simulink model "W06_Tiny_Town_cs"  (R2019a)
settings: Solver=ode5  StartTime=0.0  StopTime=inf  FixedStep=1/20  RelTol=1e-3
PreLoadFcn:
  | mbxruntime.callbacks.PreLoadFcn(bdroot);
PostLoadFcn:
  | mbxruntime.callbacks.PostLoadFcn(bdroot);
InitFcn:
  | mbxruntime.callbacks.InitFcn(bdroot);
StartFcn:
  | mbxruntime.callbacks.StartFcn(bdroot);
StopFcn:
  | mbxruntime.callbacks.StopFcn(bdroot);
model workspace: external: MAT-File .\W06_Tiny_Town_cs_hws.mat (data not in the file)
undefined symbols (not defined in the file or in its folder): DiscIntNeverNeededParam, InitImageOutputDir, mbxruntime, tabledata, W06_Tiny_Town_cs_0347f368afc477f7, W06_Tiny_Town_cs_06d739b3240d4bd1, W06_Tiny_Town_cs_0f8ec0220805dc92, W06_Tiny_Town_cs_158eea2914cd8c14, W06_Tiny_Town_cs_18b17a0c58606dc8, W06_Tiny_Town_cs_19806d8538d6bb90, W06_Tiny_Town_cs_1ceb610c831ebc6c, W06_Tiny_Town_cs_24c71a941f2399ee, W06_Tiny_Town_cs_28d17e17e50ff375, W06_Tiny_Town_cs_29e44574efa0e72f, W06_Tiny_Town_cs_2ebfd9727ae5049f, W06_Tiny_Town_cs_3b9dd96920beca23, W06_Tiny_Town_cs_4a5ba1a10aa72aa4, W06_Tiny_Town_cs_4b7992cae6b11fea, W06_Tiny_Town_cs_4ce1089559374df3, W06_Tiny_Town_cs_4f1eca6f5670696f, W06_Tiny_Town_cs_56de7514e81a64a4, W06_Tiny_Town_cs_5815099e4ab8d5b1, W06_Tiny_Town_cs_59a193f7803a15f8, W06_Tiny_Town_cs_5a93c0b4041e538b, W06_Tiny_Town_cs_5e22ff2291c0d8f8, W06_Tiny_Town_cs_664a4c8dcb6e1d77, W06_Tiny_Town_cs_66e74ff0a825ce8c, W06_Tiny_Town_cs_6f6fc115e33636b9, W06_Tiny_Town_cs_762b24f74e6359cd, W06_Tiny_Town_cs_7e7dfe0ad6d20cde, W06_Tiny_Town_cs_8dbb769f58f1ae22, W06_Tiny_Town_cs_9732a70429881892, W06_Tiny_Town_cs_97e2037932c1d396, W06_Tiny_Town_cs_99e9b9fe56cd6c11, W06_Tiny_Town_cs_9d4b19fadf9db3f5, W06_Tiny_Town_cs_9e5d5712939b904c, W06_Tiny_Town_cs_9fe5ad465f6cdbf3, W06_Tiny_Town_cs_a263437ac60b94d3, W06_Tiny_Town_cs_a313ed4746bdbf42, W06_Tiny_Town_cs_a3bc7bd64557c06d, W06_Tiny_Town_cs_af25170a5cd54ac4, W06_Tiny_Town_cs_b0bfde99f178c69e, W06_Tiny_Town_cs_b828188f0394b7ed, W06_Tiny_Town_cs_b8ac5a8063403724, W06_Tiny_Town_cs_c0c1ce03c301d04b, W06_Tiny_Town_cs_c5d7b9713d9c4410, W06_Tiny_Town_cs_cce5d3f0bd4fe0dd, W06_Tiny_Town_cs_d4161cd6ae7b274e, W06_Tiny_Town_cs_d7f1a2863608ebc5, W06_Tiny_Town_cs_e07aed9c56d02b7c, W06_Tiny_Town_cs_e4fcf49468faab60, W06_Tiny_Town_cs_e81ada3a1b2b4b0f, W06_Tiny_Town_cs_f328760c8f041e3e, W06_Tiny_Town_cs_fbbe35eb7fc27d63, W06_Tiny_Town_cs_fe7173e9daa72ca4, W06_Tiny_Town_cs_Female_Regular_1_Path_pathUniqueID, W06_Tiny_Town_cs_Ford_Focus_Stationwagon_2_Path_pathUniqueID, W06_Tiny_Town_cs_Nissan_Cabstar_Boxtruck_1_Path_pathUniqueID
libraries: adeye_lib x38, PreScanSimulinkLibrary x16, simulink x4, simulink_extras x3, robotlib x1, PreScanUsefulBlocks x1
(part 2 of 8)

== system W06_Tiny_Town_cs/ANIM_Child_Regular_1 ==
  ANIM_Child_Regular_1 : Inport  Tag=inport/AnimationOutport  OutDataTypeStr=Bus: PRESCAN_ANIMACTUATORDATA  PortDimensions=1  SampleTime=1/20  BusOutputAsStruct=on
  Actuator : S-Function  FunctionName=sfun_AnimActuator  Parameters=UniqueID, TimeStep  SFunctionDeploymentMode=off  EnableBusSupport=off  mask(PreScan Sink Block: State Animation){UniqueID=28581, TimeStep=1/20}
      mask prompts: UniqueID "Auto-Assigned: Unique ID"; TimeStep "Auto-Assigned: Upload Period [s]"
      mask help: The Human Animation port allows the human to walk, run or bend
      mask Help: eval('openHelp(239)')
      mask Display: image(imread('HumanAnimated.jpg'))
  wires:
  ANIM_Child_Regular_1/1 -> Actuator/1

== system W06_Tiny_Town_cs/ANIM_Female_Regular_1 ==
  ANIM_Female_Regular_1 : Inport  Tag=inport/AnimationOutport  OutDataTypeStr=Bus: PRESCAN_ANIMACTUATORDATA  PortDimensions=1  SampleTime=1/20  BusOutputAsStruct=on
  Actuator : S-Function  FunctionName=sfun_AnimActuator  Parameters=UniqueID, TimeStep  SFunctionDeploymentMode=off  EnableBusSupport=off  mask(PreScan Sink Block: State Animation){UniqueID=28708, TimeStep=1/20}
      mask prompts: UniqueID "Auto-Assigned: Unique ID"; TimeStep "Auto-Assigned: Upload Period [s]"
      mask help: The Human Animation port allows the human to walk, run or bend
      mask Help: eval('openHelp(239)')
      mask Display: image(imread('HumanAnimated.jpg'))
  wires:
  ANIM_Female_Regular_1/1 -> Actuator/1

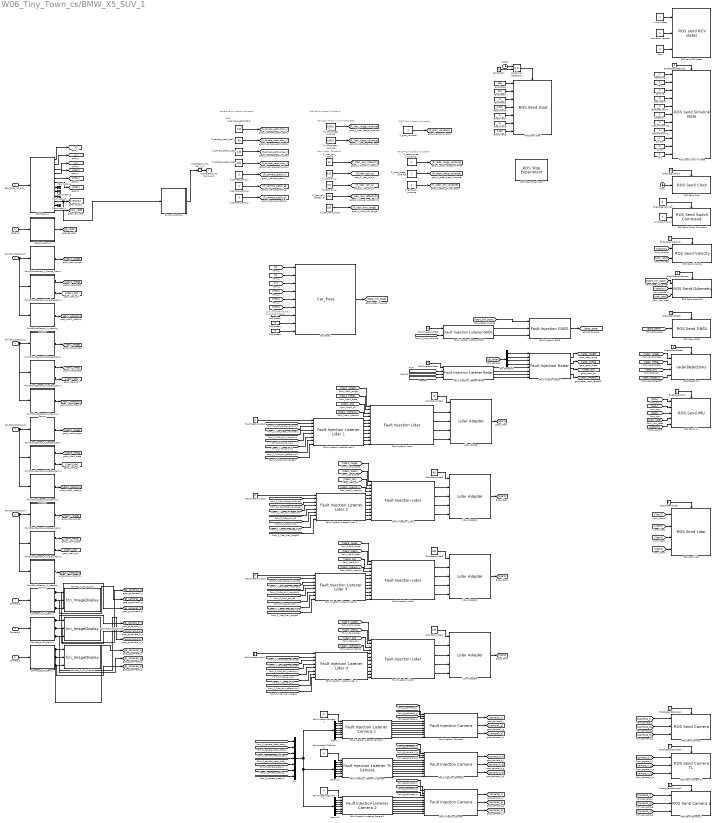
== system W06_Tiny_Town_cs/BMW_X5_SUV_1 ==
  note: CoG  compared
      | to the backwheels
      | center
  note: Gaussian random noise, Parameters
  note: Radar Fault Injection Constants
  note: GNSS Fault Injection Constants
  note: Rain model, Constants
  note: Lidar Fault injection Constants
  note: Patch
  note: Camera Fault injection Constants
  SELF_BMW_X5_SUV_1 : Inport  Tag=inport/SelfPort  OutDataTypeStr=Bus: PRESCAN_SELFSENSORDATA  PortDimensions=1  SampleTime=1/20  BusOutputAsStruct=on
  Radar_1 : Inport  Tag=inport/Radar  Port=2  OutDataTypeStr=Bus: PRESCAN_SCANNERSENSOR_MESSAGE  PortDimensions=7  SampleTime=1/20  BusOutputAsStruct=on
  PointCloudSensor_1 : Inport  Tag=inport/PointCloudInport  Port=3  OutDataTypeStr=single  SampleTime=1/20  BusOutputAsStruct=on
  PointCloudSensor_2 : Inport  Tag=inport/PointCloudInport  Port=4  OutDataTypeStr=single  SampleTime=1/20  BusOutputAsStruct=on
  PointCloudSensor_3 : Inport  Tag=inport/PointCloudInport  Port=5  OutDataTypeStr=single  SampleTime=1/20  BusOutputAsStruct=on
  PointCloudSensor_4 : Inport  Tag=inport/PointCloudInport  Port=6  OutDataTypeStr=single  SampleTime=1/20  BusOutputAsStruct=on
  Camera_1 : Inport  Tag=inport/Camera/CameraSensor  Port=7  OutDataTypeStr=uint8  SampleTime=1/20  BusOutputAsStruct=on
  Camera_tl : Inport  Tag=inport/Camera/CameraSensor  Port=8  OutDataTypeStr=uint8  SampleTime=1/20  BusOutputAsStruct=on
  Camera_2 : Inport  Tag=inport/Camera/CameraSensor  Port=9  OutDataTypeStr=uint8  SampleTime=1/20  BusOutputAsStruct=on
  Activation request : Constant  OutDataTypeStr=Inherit: Inherit via back propagation
  Bus Selector1 : BusSelector  OutputSignals=Range[m],Theta[deg],Phi[deg],TargetTypeID[-]
  Camera_1_CM_Demux : Subsystem  Tag=demux/Camera/Color  mask{SensorName=Camera_1, hres=960, vres=720}
      mask prompts: SensorName "Sensor Name"; hres "Horizontal Resolution"; vres "Vertical Resolution"
      mask Help: eval('openHelp(457)')
      mask Display:
      | fprintf('MONO CAMERA:\n Color\n %s \n %d x %d px',SensorName,hres,vres)
      | port_label('output',1,'R')
      | port_label('output',2,'G')
      | port_label('output',3,'B')
  Camera_1_CM_Display : M-S-Function  Tag=CameraSensor_Color_Display  InitFcn=InitImageOutputDir(gcb);  FunctionName=fcn_ImageDisplay  Parameters=SensorName EnableDisplay EnablePosition DisplayPosition FigureHandle SaveResults BitmapFormat TempOutputDir CameraType DataType  mask(PreScan Color Display Block){SensorName=Camera_1, EnableDisplay=off, EnablePosition=off, DisplayPosition=[10 10 960 720], FigureHandle=2792805, SaveResults=off, Format=PNG, TempOutputDir=0, CameraType=Mono, DataType=uint8}
      mask prompts: SensorName "User Specified: Title of Display"; EnableDisplay "Active"; EnablePosition "Set Display window position"; DisplayPosition "Display window position [xpos ypos width height]"; FigureHandle "Unique Handle"; SaveResults "Save results"; TempOutputDir "OutputDir"; CameraType "Camera Type"; DataType "Image Data Type"
      mask help: This block displays the RGB output of a PreScan camera sensor.
      mask init:
      | if EnableDisplay
      |     EnableString='';
      |     EnableColor='gray';
      | else
      |     EnableString='INACTIVE';
      |     EnableColor='red';
      | end
      | switch Format
      |     case 1
      |         BitmapFormat = 'png';
      |     case 2
      |         BitmapFormat = 'bmp';
      |     case 3
      |         BitmapFormat = 'jpg';
      | end 
      | if CameraType==1
      |     CameraTypeName='MONO';
      |     PortNumber=0;
      | else
      |     CameraTypeName='STEREO';
      |     PortNumber=3;
      | end
      settings: CopyFcn=CopyFcnDisplay  DeleteFcn=PreScanBlockDeleteFcn;  ModelCloseFcn=fcn_ImageDisplay_ModelCloseFcn
      mask Help: eval('openHelp(457)')
      mask Callback EnablePosition:
      | MV=get_param(gcb,'MaskVisibilities');
      | if strcmp(get_param(gcb,'EnablePosition'),'on')
      |     MV{4}='on';
      | else
      |     MV{4}='off';
      | end
      | set_param(gcb,'MaskVisibilities',MV);
      | clear MV;
      mask TypeOptions Format: PNG | BMP | JPG
      mask TypeOptions CameraType: Mono | Stereo
      mask TypeOptions DataType: uint8 | single
      mask Display:
      | color(EnableColor);
      | fprintf('%s\n DISPLAY:\n Color \n %s',EnableString,SensorName)
      | port_label('input',1,'R')
      | port_label('input',2,'G')
      | port_label('input',3,'B')
      | port_label('input',PortNumber+1,'R')
      | port_label('input',PortNumber+2,'G')
      | port_label('input',PortNumber+3,'B')
  Camera_2_CM_Demux : Subsystem  Tag=demux/Camera/Color  mask{SensorName=Camera_2, hres=960, vres=720}
      mask prompts: SensorName "Sensor Name"; hres "Horizontal Resolution"; vres "Vertical Resolution"
      mask Help: eval('openHelp(457)')
      mask Display:
      | fprintf('MONO CAMERA:\n Color\n %s \n %d x %d px',SensorName,hres,vres)
      | port_label('output',1,'R')
      | port_label('output',2,'G')
      | port_label('output',3,'B')
  Camera_2_CM_Display : M-S-Function  Tag=CameraSensor_Color_Display  InitFcn=InitImageOutputDir(gcb);  FunctionName=fcn_ImageDisplay  Parameters=SensorName EnableDisplay EnablePosition DisplayPosition FigureHandle SaveResults BitmapFormat TempOutputDir CameraType DataType  mask(PreScan Color Display Block){SensorName=Camera_2, EnableDisplay=off, EnablePosition=off, DisplayPosition=[10 10 960 720], FigureHandle=2792807, SaveResults=off, Format=PNG, TempOutputDir=0, CameraType=Mono, DataType=uint8}
      mask prompts: SensorName "User Specified: Title of Display"; EnableDisplay "Active"; EnablePosition "Set Display window position"; DisplayPosition "Display window position [xpos ypos width height]"; FigureHandle "Unique Handle"; SaveResults "Save results"; TempOutputDir "OutputDir"; CameraType "Camera Type"; DataType "Image Data Type"
      mask help: This block displays the RGB output of a PreScan camera sensor.
      mask init: same as W06_Tiny_Town_cs/BMW_X5_SUV_1/Camera_1_CM_Display
      settings: CopyFcn=CopyFcnDisplay  DeleteFcn=PreScanBlockDeleteFcn;  ModelCloseFcn=fcn_ImageDisplay_ModelCloseFcn
      mask Help: eval('openHelp(457)')
      mask Callback EnablePosition:
      | MV=get_param(gcb,'MaskVisibilities');
      | if strcmp(get_param(gcb,'EnablePosition'),'on')
      |     MV{4}='on';
      | else
      |     MV{4}='off';
      | end
      | set_param(gcb,'MaskVisibilities',MV);
      | clear MV;
      mask TypeOptions Format: PNG | BMP | JPG
      mask TypeOptions CameraType: Mono | Stereo
      mask TypeOptions DataType: uint8 | single
      mask Display:
      | color(EnableColor);
      | fprintf('%s\n DISPLAY:\n Color \n %s',EnableString,SensorName)
      | port_label('input',1,'R')
      | port_label('input',2,'G')
      | port_label('input',3,'B')
      | port_label('input',PortNumber+1,'R')
      | port_label('input',PortNumber+2,'G')
      | port_label('input',PortNumber+3,'B')
  Camera_tl_CM_Demux : Subsystem  Tag=demux/Camera/Color  mask{SensorName=Camera_tl, hres=960, vres=720}
      mask prompts: SensorName "Sensor Name"; hres "Horizontal Resolution"; vres "Vertical Resolution"
      mask Help: eval('openHelp(457)')
      mask Display:
      | fprintf('MONO CAMERA:\n Color\n %s \n %d x %d px',SensorName,hres,vres)
      | port_label('output',1,'R')
      | port_label('output',2,'G')
      | port_label('output',3,'B')
  Camera_tl_CM_Display : M-S-Function  Tag=CameraSensor_Color_Display  InitFcn=InitImageOutputDir(gcb);  FunctionName=fcn_ImageDisplay  Parameters=SensorName EnableDisplay EnablePosition DisplayPosition FigureHandle SaveResults BitmapFormat TempOutputDir CameraType DataType  mask(PreScan Color Display Block){SensorName=Camera_tl, EnableDisplay=off, EnablePosition=off, DisplayPosition=[10 10 960 720], FigureHandle=2792806, SaveResults=off, Format=PNG, TempOutputDir=0, CameraType=Mono, DataType=uint8}
      mask prompts: SensorName "User Specified: Title of Display"; EnableDisplay "Active"; EnablePosition "Set Display window position"; DisplayPosition "Display window position [xpos ypos width height]"; FigureHandle "Unique Handle"; SaveResults "Save results"; TempOutputDir "OutputDir"; CameraType "Camera Type"; DataType "Image Data Type"
      mask help: This block displays the RGB output of a PreScan camera sensor.
      mask init: same as W06_Tiny_Town_cs/BMW_X5_SUV_1/Camera_1_CM_Display
      settings: CopyFcn=CopyFcnDisplay  DeleteFcn=PreScanBlockDeleteFcn;  ModelCloseFcn=fcn_ImageDisplay_ModelCloseFcn
      mask Help: eval('openHelp(457)')
      mask Callback EnablePosition:
      | MV=get_param(gcb,'MaskVisibilities');
      | if strcmp(get_param(gcb,'EnablePosition'),'on')
      |     MV{4}='on';
      | else
      |     MV{4}='off';
      | end
      | set_param(gcb,'MaskVisibilities',MV);
      | clear MV;
      mask TypeOptions Format: PNG | BMP | JPG
      mask TypeOptions CameraType: Mono | Stereo
      mask TypeOptions DataType: uint8 | single
      mask Display:
      | color(EnableColor);
      | fprintf('%s\n DISPLAY:\n Color \n %s',EnableString,SensorName)
      | port_label('input',1,'R')
      | port_label('input',2,'G')
      | port_label('input',3,'B')
      | port_label('input',PortNumber+1,'R')
      | port_label('input',PortNumber+2,'G')
      | port_label('input',PortNumber+3,'B')
  Car_Pose1 : adeye_lib/Car_Pose  SystemSampleTime=-1
  Clock : Clock
  Clock2 : Clock
  CoG offset x : Constant  Value=0
  CoG offset y : Constant  Value=0
  CoG offset z : Constant  Value=0
  Constant27 : Constant  Value=0
  Demux : Demux  Outputs=7
  Demux1 : Demux  Outputs=7
  Demux2 : Demux  Outputs=7
  Detection : Constant
  Dynamics_Empty : Subsystem  Tag=Dynamics_Empty
      mask Help: eval('openHelp(202)')
      mask Display: port_label('output', 1, 'State');text(0,0,' Empty\n')
  EnableSendCamera1 : Constant  OutDataTypeStr=Inherit: Inherit via back propagation
  EnableSendCamera2 : Constant  OutDataTypeStr=Inherit: Inherit via back propagation
  EnableSendCameraTL : Constant  OutDataTypeStr=Inherit: Inherit via back propagation
  EnableSendClock : Constant  OutDataTypeStr=Inherit: Inherit via back propagation
  EnableSendFeatures : Constant  Value=0  OutDataTypeStr=Inherit: Inherit via back propagation
  EnableSendGNSS : Constant  OutDataTypeStr=Inherit: Inherit via back propagation
  EnableSendIMU : Constant  OutDataTypeStr=Inherit: Inherit via back propagation
  EnableSendLidar : Constant  OutDataTypeStr=Inherit: Inherit via back propagation
  EnableSendOdometry : Constant
  EnableSendRadar : Constant  OutDataTypeStr=Inherit: Inherit via back propagation
  EnableSendSwitch : Constant  Value=0  OutDataTypeStr=Inherit: Inherit via back propagation  SampleTime=0.05
  EnableSendVelocity : Constant  OutDataTypeStr=Inherit: Inherit via back propagation
  FakeLocalization : Constant
  Fault : Constant  Value=0  OutDataTypeStr=Inherit: Inherit via back propagation
  Fault Injection Camera : adeye_lib/Fault Injection Camera  idy=200  idx=100  x=100  y=150  R=0  G=0  B=0
  Fault Injection Camera1 : adeye_lib/Fault Injection Camera  idy=200  idx=100  x=100  y=150  R=0  G=0  B=0
  Fault Injection Camera2 : adeye_lib/Fault Injection Camera  idy=200  idx=100  x=100  y=150  R=0  G=0  B=0
  Fault Injection GNSS : adeye_lib/Fault Injection GNSS  f=20
  Fault Injection Lidar{,1..3} (4 alike) : adeye_lib/Fault Injection Lidar  f=20  p=225*16
  Fault Injection Listener Camera 1 : adeye_lib/Fault Injection Listener Camera 1  SystemSampleTime=-1
  Fault Injection Listener Camera 2 : adeye_lib/Fault Injection Listener Camera 2  SystemSampleTime=-1
  Fault Injection Listener GNSS : adeye_lib/Fault Injection Listener GNSS  SystemSampleTime=-1
  Fault Injection Listener Lidar 1 : adeye_lib/Fault Injection Listener Lidar 1  SystemSampleTime=-1
  Fault Injection Listener Lidar 2 : adeye_lib/Fault Injection Listener Lidar 2  SystemSampleTime=-1
  Fault Injection Listener Lidar 3 : adeye_lib/Fault Injection Listener Lidar 3  SystemSampleTime=-1
  Fault Injection Listener Lidar 4 : adeye_lib/Fault Injection Listener Lidar 4  SystemSampleTime=-1
  Fault Injection Listener Radar : adeye_lib/Fault Injection Listener Radar  SystemSampleTime=-1
  Fault Injection Listener TL Camera : adeye_lib/Fault Injection Listener TL Camera  SystemSampleTime=-1
  Fault Injection Radar : adeye_lib/Fault Injection Radar  n=7
  FaultInjectionCamera1 : Constant  Value=0
  FaultInjectionCamera2 : Constant  Value=0
  FaultInjectionGNSS : Constant  Value=0  OutDataTypeStr=Inherit: Inherit via back propagation  SampleTime=0.05
  FaultInjectionLidar{1..4} (4 alike) : Constant  Value=0  OutDataTypeStr=Inherit: Inherit via back propagation
  FaultInjectionRadar : Constant  Value=0
  FaultInjectionTLCamera : Constant  Value=0
  GoalOrientW : Constant  Value=0.707
  GoalOrientX : Constant  Value=0
  GoalOrientY : Constant  Value=0
  GoalOrientZ : Constant  Value=0.707
  GoalPoseX : Constant  Value=183
  GoalPoseY : Constant  Value=111
  GoalPoseZ : Constant  Value=0
  Initial checks : Constant  OutDataTypeStr=Inherit: Inherit via back propagation
  Lidar Adapter{,1..3} (4 alike) : adeye_lib/Lidar Adapter  SystemSampleTime=-1
  Localization : Constant  Value=0
  Map : Constant
  MissionPlanning : Constant
  MotionPlanning : Constant
  Mux : Mux  Inputs=7
  OrientationLidar1 : Constant  Value=0  OutDataTypeStr=Inherit: Inherit via back propagation
  OrientationLidar2 : Constant  Value=90  OutDataTypeStr=Inherit: Inherit via back propagation
  OrientationLidar3 : Constant  Value=180  OutDataTypeStr=Inherit: Inherit via back propagation
  OrientationLidar4 : Constant  Value=270  OutDataTypeStr=Inherit: Inherit via back propagation
  PointCloudSensor_1_Angles_Demux : Subsystem  Tag=demux/PCS/Angles  mask{SensorName=PointCloudSensor_1, offset=225, hres=225, vres=16}
      mask prompts: SensorName "Sensor Name"; offset "Data Start"; hres "Horizontal Resolution"; vres "Vertical Resolution"
      mask Help: eval('openHelp(6400)')
      mask Display:
      | fprintf('Point Cloud:\n Data\n %s \n %d x %d px',SensorName,hres,vres)
      | port_label('output',1,'Theta')
      | port_label('output',2,'Phi')
  PointCloudSensor_1_Intensity_Demux : Subsystem  Tag=demux/PCS/Intensity  mask{SensorName=PointCloudSensor_1, offset=675, hres=225, vres=16}
      mask prompts: SensorName "Sensor Name"; offset "Data Start"; hres "Horizontal Resolution"; vres "Vertical Resolution"
      mask Help: eval('openHelp(6400)')
      mask Display:
      | fprintf('Point Cloud:\n Data\n %s \n %d x %d px',SensorName,hres,vres)
      | port_label('output',1,'Intensity')
  PointCloudSensor_1_Range_Demux : Subsystem  Tag=demux/PCS/Range  mask{SensorName=PointCloudSensor_1, offset=0, hres=225, vres=16}
      mask prompts: SensorName "Sensor Name"; offset "Data Start"; hres "Horizontal Resolution"; vres "Vertical Resolution"
      mask Help: eval('openHelp(6400)')
      mask Display:
      | fprintf('Point Cloud:\n Data\n %s \n %d x %d px',SensorName,hres,vres)
      | port_label('output',1,'Range')
  PointCloudSensor_2_Angles_Demux : Subsystem  Tag=demux/PCS/Angles  mask{SensorName=PointCloudSensor_2, offset=225, hres=225, vres=16}
      mask prompts: SensorName "Sensor Name"; offset "Data Start"; hres "Horizontal Resolution"; vres "Vertical Resolution"
      mask Help: eval('openHelp(6400)')
      mask Display:
      | fprintf('Point Cloud:\n Data\n %s \n %d x %d px',SensorName,hres,vres)
      | port_label('output',1,'Theta')
      | port_label('output',2,'Phi')
  PointCloudSensor_2_Intensity_Demux : Subsystem  Tag=demux/PCS/Intensity  mask{SensorName=PointCloudSensor_2, offset=675, hres=225, vres=16}
      mask prompts: SensorName "Sensor Name"; offset "Data Start"; hres "Horizontal Resolution"; vres "Vertical Resolution"
      mask Help: eval('openHelp(6400)')
      mask Display:
      | fprintf('Point Cloud:\n Data\n %s \n %d x %d px',SensorName,hres,vres)
      | port_label('output',1,'Intensity')
  PointCloudSensor_2_Range_Demux : Subsystem  Tag=demux/PCS/Range  mask{SensorName=PointCloudSensor_2, offset=0, hres=225, vres=16}
      mask prompts: SensorName "Sensor Name"; offset "Data Start"; hres "Horizontal Resolution"; vres "Vertical Resolution"
      mask Help: eval('openHelp(6400)')
      mask Display:
      | fprintf('Point Cloud:\n Data\n %s \n %d x %d px',SensorName,hres,vres)
      | port_label('output',1,'Range')
  PointCloudSensor_3_Angles_Demux : Subsystem  Tag=demux/PCS/Angles  mask{SensorName=PointCloudSensor_3, offset=225, hres=225, vres=16}
      mask prompts: SensorName "Sensor Name"; offset "Data Start"; hres "Horizontal Resolution"; vres "Vertical Resolution"
      mask Help: eval('openHelp(6400)')
      mask Display:
      | fprintf('Point Cloud:\n Data\n %s \n %d x %d px',SensorName,hres,vres)
      | port_label('output',1,'Theta')
      | port_label('output',2,'Phi')
  PointCloudSensor_3_Intensity_Demux : Subsystem  Tag=demux/PCS/Intensity  mask{SensorName=PointCloudSensor_3, offset=675, hres=225, vres=16}
      mask prompts: SensorName "Sensor Name"; offset "Data Start"; hres "Horizontal Resolution"; vres "Vertical Resolution"
      mask Help: eval('openHelp(6400)')
      mask Display:
      | fprintf('Point Cloud:\n Data\n %s \n %d x %d px',SensorName,hres,vres)
      | port_label('output',1,'Intensity')
  PointCloudSensor_3_Range_Demux : Subsystem  Tag=demux/PCS/Range  mask{SensorName=PointCloudSensor_3, offset=0, hres=225, vres=16}
      mask prompts: SensorName "Sensor Name"; offset "Data Start"; hres "Horizontal Resolution"; vres "Vertical Resolution"
      mask Help: eval('openHelp(6400)')
      mask Display:
      | fprintf('Point Cloud:\n Data\n %s \n %d x %d px',SensorName,hres,vres)
      | port_label('output',1,'Range')
  PointCloudSensor_4_Angles_Demux : Subsystem  Tag=demux/PCS/Angles  mask{SensorName=PointCloudSensor_4, offset=225, hres=225, vres=16}
      mask prompts: SensorName "Sensor Name"; offset "Data Start"; hres "Horizontal Resolution"; vres "Vertical Resolution"
      mask Help: eval('openHelp(6400)')
      mask Display:
      | fprintf('Point Cloud:\n Data\n %s \n %d x %d px',SensorName,hres,vres)
      | port_label('output',1,'Theta')
      | port_label('output',2,'Phi')
  PointCloudSensor_4_Intensity_Demux : Subsystem  Tag=demux/PCS/Intensity  mask{SensorName=PointCloudSensor_4, offset=675, hres=225, vres=16}
      mask prompts: SensorName "Sensor Name"; offset "Data Start"; hres "Horizontal Resolution"; vres "Vertical Resolution"
      mask Help: eval('openHelp(6400)')
      mask Display:
      | fprintf('Point Cloud:\n Data\n %s \n %d x %d px',SensorName,hres,vres)
      | port_label('output',1,'Intensity')
  PointCloudSensor_4_Range_Demux : Subsystem  Tag=demux/PCS/Range  mask{SensorName=PointCloudSensor_4, offset=0, hres=225, vres=16}
      mask prompts: SensorName "Sensor Name"; offset "Data Start"; hres "Horizontal Resolution"; vres "Vertical Resolution"
      mask Help: eval('openHelp(6400)')
      mask Display:
      | fprintf('Point Cloud:\n Data\n %s \n %d x %d px',SensorName,hres,vres)
      | port_label('output',1,'Range')
  ROS Send Camera : adeye_lib/ROS Send Camera  SystemSampleTime=-1
  ROS Send Camera 2 : adeye_lib/ROS Send Camera 2  SystemSampleTime=-1
  ROS Send Camera TL : adeye_lib/ROS Send Camera TL  SystemSampleTime=-1
  ROS Send Clock : adeye_lib/ROS Send Clock  SystemSampleTime=-1
  ROS Send GNSS : adeye_lib/ROS Send GNSS  SystemSampleTime=-1
  ROS Send Goal : adeye_lib/ROS Send Goal  SystemSampleTime=-1
  ROS Send IMU : adeye_lib/ROS Send IMU  SystemSampleTime=-1
  ROS Send Lidar : adeye_lib/ROS Send Lidar  SystemSampleTime=-1
  ROS Send Odometry : adeye_lib/ROS Send Odometry  SystemSampleTime=-1
  ROS Send Simulink State : adeye_lib/ROS Send Simulink State  SystemSampleTime=-1
  ROS Send Switch Command : adeye_lib/ROS Send Switch Command  SystemSampleTime=-1
  ROS Send Velocity : adeye_lib/ROS Send Velocity  SystemSampleTime=-1
  "ROS Stop Experiment " : adeye_lib/ROS Stop Experiment  SystemSampleTime=-1
  ROS send RCV states : adeye_lib/ROS send RCV states  SystemSampleTime=-1
  Radar_1_Demux : Subsystem  Tag=demux/Radar  TreatAsAtomicUnit=on  mask(PreScan Demux Block: Radar){MAXMESSAGES=7}
      mask prompts: MAXMESSAGES "Number of Objects"
      mask help:
      | The Radar Sensor is a detailed sensor based on a physical radar
      | model that includes Antenna GAIN Maps (AGM) and atmospheric
      | attenuation.
      |
      | For more information, please click Help.
      mask Help: eval('openHelp(1464)')
      mask Display:
      | port_label('input',1,'Radar')
      | port_label('output',1,'Radar Data')
  Recording : Constant
  Relational Operator1 : RelationalOperator  Operator===  OutDataTypeStr=boolean  RndMeth=Simplest
  Rviz : Constant
  SELF_Demux : Subsystem  Tag=demux/SelfPort  mask(PreScan Demux Block:){}
      mask help:
      | The SELF port shows (state) information of the actor itself. The outputs are position in the experiment's axis system and the GPS coordinates, and the object's absolute velocity and compass heading.
      |
      | For more information, please click Help.
      settings: DeleteFcn=PreScanBlockDeleteFcn;
      mask Help: eval('openHelp(462)')
      mask Display:
      | port_label('output',1,'x [m]')
      | port_label('output',2,'y [m]')
      | port_label('output',3,'z [m]','texmode','on')
      | port_label('output',4,'Rotx [deg]','texmode','on')
      | port_label('output',5,'Roty [deg]','texmode','on')
      | port_label('output',6,'Rotz [deg]','texmode','on')
      | port_label('output',7,'GPS lat [deg]','texmode','on')
      | port_label('output',8,'GPS long [deg]','texmode','on')
      | port_label('output',9,'GPS alt [m]','texmode','on')
      | port_label('output',10,'Velocity [m/s]')
      | port_label('output',11,'Heading [deg]')
      | port_label('output',12,'Yaw rate [deg/s]')
  STATE_BMW_X5_SUV_1_rc : RateTransition  Tag=mux_rc/StatePort  OutPortSampleTimeOpt=Inherit
  Sensing : Constant
  Ssmp : Constant
  Switch : Constant
  SwitchCommand : Constant  OutDataTypeStr=Inherit: Inherit via back propagation  SampleTime=0.05
  Terminator_{1..4} (4 alike) : Terminator
  fi_camera_patch_b : Constant  Value=0
  fi_camera_patch_g : Constant  Value=0
  fi_camera_patch_r : Constant  Value=0
  fi_camera_patch_size_x : Constant  Value=100
  fi_camera_patch_size_y : Constant  Value=100
  fi_camera_patch_start_x : Constant  Value=110
  fi_camera_patch_start_y : Constant  Value=50
  fi_gnss_variance : Constant
  fi_lidar_max_range : Constant  Value=150
  fi_lidar_rain_a : Constant  Value=0.01
  fi_lidar_rain_b : Constant  Value=0.6
  fi_lidar_rain_intensity : Constant  Value=20
  fi_lidar_rain_reflectivity : Constant  Value=0.9
  fi_lidar_range_variance : Constant  Value=0.0001
  fi_lidar_theta_variance : Constant  Value=0.0001
  fi_radar_phi_variance : Constant
  fi_radar_range_variance : Constant
  fi_radar_theta_variance : Constant
  radarDetections : adeye_lib/radarDetections  SystemSampleTime=-1
  STATE_BMW_X5_SUV_1_bus : Outport  Tag=outport/StatePort  OutDataTypeStr=Bus: PRESCAN_STATEACTUATORDATA  PortDimensions=1  SampleTime=1/20
  wires:
  GoalOrientZ/1 -> ROS Send Goal/7
  GoalOrientW/1 -> ROS Send Goal/4
  GoalOrientX/1 -> ROS Send Goal/5
  GoalOrientY/1 -> ROS Send Goal/6
  GoalPoseX/1 -> ROS Send Goal/1
  GoalPoseY/1 -> ROS Send Goal/2
  GoalPoseZ/1 -> ROS Send Goal/3
  Constant27/1 -> Relational Operator1/2
  Relational Operator1/1 -> ROS Send Goal/Enable
  Clock2/1 -> Relational Operator1/1
  Demux1/2 -> Fault Injection Listener TL Camera/3
  fi_lidar_range_variance/1 -> [fi_lidar_range_variance]
  Fault Injection Listener Radar/2 -> Fault Injection Radar/6
  [Rotx] -> ROS Send IMU/1
  [lidar1_theta] -> Fault Injection Lidar/2
  Fault Injection Listener TL Camera/1 -> Fault Injection Camera2/4
  Demux/1 -> Fault Injection Listener Camera 1/2
  [gt_camera1_r] -> Fault Injection Camera1/1
  [fi_lidar_rain_reflectivity] -> Fault Injection Listener Lidar 4/7
  Fault Injection Lidar2/4 -> Lidar Adapter2/5
  Demux2/3 -> Fault Injection Listener Camera 2/4
  Mux/1 -> Demux2/1, Demux1/1, Demux/1
  Demux1/3 -> Fault Injection Listener TL Camera/4
  [lidar4_phi] -> Fault Injection Lidar3/3
  [fi_lidar_rain_b] -> Fault Injection Listener Lidar 3/6
  [gt_camera_tl_g] -> Fault Injection Camera2/2
  Fault Injection Radar/2 -> [radar_theta]
  Demux1/7 -> Fault Injection Listener TL Camera/8
  Fault Injection Camera2/1 -> [camera_tl_r]
  Demux2/7 -> Fault Injection Listener Camera 2/8
  [fi_camera_patch_size_x] -> Mux/3
  Fault Injection Camera1/3 -> [camera1_b]
  Demux/2 -> Fault Injection Listener Camera 1/3
  [fi_gnss_variance] -> Fault Injection Listener GNSS/2
  Demux/4 -> Fault Injection Listener Camera 1/5
  Fault Injection Listener Lidar 4/1 -> Fault Injection Lidar3/5
  OrientationLidar1/1 -> Lidar Adapter/1
  Fault Injection Listener Lidar 3/5 -> Fault Injection Lidar2/9
  Fault Injection Camera2/2 -> [camera_tl_g]
  Fault Injection Listener Lidar 4/2 -> Fault Injection Lidar3/6
  Demux/3 -> Fault Injection Listener Camera 1/4
  Demux1/1 -> Fault Injection Listener TL Camera/2
  Fault Injection Listener Lidar 2/8 -> Fault Injection Lidar1/12
  [camera_tl_r] -> ROS Send Camera TL/1
  Activation request/1 -> ROS send RCV states/2
  [fi_camera_patch_g] -> Mux/6
  Demux/7 -> Fault Injection Listener Camera 1/8
  fi_lidar_theta_variance/1 -> [fi_lidar_theta_variance]
  [fi_lidar_range_variance] -> Fault Injection Listener Lidar 2/2
  EnableSendIMU/1 -> ROS Send IMU/Enable
  Fault Injection Listener TL Camera/7 -> Fault Injection Camera2/10
  Demux2/2 -> Fault Injection Listener Camera 2/3
  Demux2/5 -> Fault Injection Listener Camera 2/6
  [fi_lidar_rain_reflectivity] -> Fault Injection Listener Lidar 1/7
  fi_camera_patch_b/1 -> [fi_camera_patch_b]
  Demux1/5 -> Fault Injection Listener TL Camera/6
  [fi_lidar_theta_variance] -> Fault Injection Listener Lidar 3/3
  Fault Injection Listener Lidar 1/1 -> Fault Injection Lidar/5
  fi_camera_patch_g/1 -> [fi_camera_patch_g]
  OrientationLidar4/1 -> Lidar Adapter3/1
  [fi_camera_patch_start_y] -> Mux/2
  [camera2_g] -> ROS Send Camera 2/2
  [fi_lidar_rain_a] -> Fault Injection Listener Lidar 2/5
  FaultInjectionTLCamera/1 -> Fault Injection Listener TL Camera/1
  [lidar4_theta] -> Fault Injection Lidar3/2
  [fi_camera_patch_start_x] -> Mux/1
  [yaw_rate] -> ROS Send IMU/4
  fi_camera_patch_start_x/1 -> [fi_camera_patch_start_x]
  [fi_lidar_max_range] -> Fault Injection Listener Lidar 4/8
  [radar_range] -> radarDetections/1
  [fi_lidar_rain_intensity] -> Fault Injection Listener Lidar 3/4
  [fi_lidar_rain_intensity] -> Fault Injection Listener Lidar 4/4
  fi_camera_patch_size_x/1 -> [fi_camera_patch_size_x]
  [camera1_r] -> ROS Send Camera/1
  Fault Injection Listener Radar/4 -> Fault Injection Radar/8
  Fault Injection Radar/4 -> [radar_targetID]
  [camera2_r] -> ROS Send Camera 2/1
  fi_radar_phi_variance/1 -> [fi_radar_phi_variance]
  [camera1_b] -> ROS Send Camera/3
  fi_camera_patch_r/1 -> [fi_camera_patch_r]
  Fault Injection Camera1/2 -> [camera1_g]
  [fi_lidar_rain_b] -> Fault Injection Listener Lidar 2/6
  Fault Injection Camera/3 -> [camera2_b]
  [fi_lidar_max_range] -> Fault Injection Listener Lidar 3/8
  Fault Injection Lidar1/4 -> Lidar Adapter1/5
  Fault Injection Camera/2 -> [camera2_g]
  Fault Injection Listener Lidar 3/4 -> Fault Injection Lidar2/8
  Fault Injection Lidar1/2 -> Lidar Adapter1/3
  [gt_radar] -> Bus Selector1/1
  [fi_radar_phi_variance] -> Fault Injection Listener Radar/4
  [camera_tl_g] -> ROS Send Camera TL/2
  Fault Injection Listener Lidar 1/3 -> Fault Injection Lidar/7
  Fault Injection Listener Camera 2/6 -> Fault Injection Camera/9
  EnableSendCameraTL/1 -> ROS Send Camera TL/Enable
  Fault Injection Listener Radar/1 -> Fault Injection Radar/5
  [radar_theta] -> radarDetections/2
  Fault Injection Lidar3/3 -> Lidar Adapter3/4
  Fault Injection Listener Lidar 1/4 -> Fault Injection Lidar/8
  [fi_lidar_rain_b] -> Fault Injection Listener Lidar 4/6
  [radar_phi] -> radarDetections/3
  Fault Injection Listener Lidar 2/7 -> Fault Injection Lidar1/11
  [gnss_pose] -> ROS Send GNSS/1
  Fault Injection Radar/1 -> [radar_range]
  fi_lidar_max_range/1 -> [fi_lidar_max_range]
  Fault Injection Listener Lidar 1/6 -> Fault Injection Lidar/10
  [velocity] -> ROS Send IMU/5
  [camera2_b] -> ROS Send Camera 2/3
  Fault Injection Lidar3/2 -> Lidar Adapter3/3
  Fault Injection Listener Camera 2/7 -> Fault Injection Camera/10
  Fault Injection Listener Lidar 1/2 -> Fault Injection Lidar/6
  [lidar3_phi] -> Fault Injection Lidar2/3
  Fault Injection Listener Camera 2/1 -> Fault Injection Camera/4
  [lidar1_range] -> Fault Injection Lidar/1
  [fi_lidar_theta_variance] -> Fault Injection Listener Lidar 4/3
  Fault Injection Listener Camera 2/2 -> Fault Injection Camera/5
  [lidar3_range] -> Fault Injection Lidar2/1
  [lidar2_range] -> Fault Injection Lidar1/1
  [fi_camera_patch_size_y] -> Mux/4
  [lidar2_theta] -> Fault Injection Lidar1/2
  Fault Injection Listener Lidar 3/2 -> Fault Injection Lidar2/6
  fi_camera_patch_start_y/1 -> [fi_camera_patch_start_y]
  fi_gnss_variance/1 -> [fi_gnss_variance]
  [fi_camera_patch_r] -> Mux/5
  [Rotz] -> ROS Send IMU/3
  CoG offset y/1 -> Car_Pose1/8
  [fi_lidar_rain_a] -> Fault Injection Listener Lidar 4/5
  [lidar2_phi] -> Fault Injection Lidar1/3
  Fault Injection GNSS/1 -> [gnss_pose]
  [lidar2_intensity] -> Fault Injection Lidar1/4
  [lidar4_range] -> Fault Injection Lidar3/1
  [fi_radar_theta_variance] -> Fault Injection Listener Radar/3
  [gt_camera2_g] -> Fault Injection Camera/2
  [gt_camera_tl_b] -> Fault Injection Camera2/3
  Clock/1 -> ROS Send Clock/1
  Fault Injection Listener Lidar 4/3 -> Fault Injection Lidar3/7
  Fault Injection Listener TL Camera/2 -> Fault Injection Camera2/5
  Fault Injection Listener TL Camera/6 -> Fault Injection Camera2/9
  [lidar1_phi] -> Fault Injection Lidar/3
  [lidar1_intensity] -> Fault Injection Lidar/4
  Lidar Adapter1/1 -> [lidar2]
  Demux1/6 -> Fault Injection Listener TL Camera/7
  Fault Injection Listener Camera 1/4 -> Fault Injection Camera1/7
  Fault Injection Camera2/3 -> [camera_tl_b]
  [fi_lidar_max_range] -> Fault Injection Listener Lidar 1/8
  Fault Injection Listener TL Camera/8 -> Fault Injection Camera2/11
  Fault Injection Listener Camera 1/5 -> Fault Injection Camera1/8
  Fault Injection Listener Radar/3 -> Fault Injection Radar/7
  Fault Injection Lidar/1 -> Lidar Adapter/2
  Fault Injection Listener Camera 1/3 -> Fault Injection Camera1/6
  Fault Injection Radar/3 -> [radar_phi]
  [fi_radar_range_variance] -> Fault Injection Listener Radar/2
  Fault Injection Listener Camera 1/7 -> Fault Injection Camera1/10
  fi_radar_range_variance/1 -> [fi_radar_range_variance]
  EnableSendFeatures/1 -> ROS Send Simulink State/Enable
  [fi_lidar_range_variance] -> Fault Injection Listener Lidar 1/2
  Demux2/1 -> Fault Injection Listener Camera 2/2
  [fi_lidar_theta_variance] -> Fault Injection Listener Lidar 1/3
  Fault Injection Listener Lidar 4/7 -> Fault Injection Lidar3/11
  Fault Injection Listener Lidar 3/6 -> Fault Injection Lidar2/10
  Fault Injection Listener Lidar 4/8 -> Fault Injection Lidar3/12
  Fault Injection Listener Lidar 3/3 -> Fault Injection Lidar2/7
  Fault Injection Listener TL Camera/4 -> Fault Injection Camera2/7
  Fault Injection Listener Lidar 3/7 -> Fault Injection Lidar2/11
  Fault Injection Listener Camera 2/8 -> Fault Injection Camera/11
  Fault Injection Listener Lidar 3/8 -> Fault Injection Lidar2/12
  [fi_lidar_rain_intensity] -> Fault Injection Listener Lidar 1/4
  Fault Injection Listener Camera 2/5 -> Fault Injection Camera/8
  Fault Injection Listener Camera 1/8 -> Fault Injection Camera1/11
  Fault Injection Listener TL Camera/3 -> Fault Injection Camera2/6
  OrientationLidar3/1 -> Lidar Adapter2/1
  [fi_camera_patch_b] -> Mux/7
  Fault Injection Listener Camera 2/3 -> Fault Injection Camera/6
  Fault Injection Lidar1/1 -> Lidar Adapter1/2
  Fault Injection Listener Lidar 2/4 -> Fault Injection Lidar1/8
  SwitchCommand/1 -> ROS Send Switch Command/1
  FaultInjectionLidar2/1 -> Fault Injection Listener Lidar 2/1
  [fi_lidar_range_variance] -> Fault Injection Listener Lidar 4/2
  Map/1 -> ROS Send Simulink State/2
  Demux/5 -> Fault Injection Listener Camera 1/6
  Fault Injection Listener Lidar 2/3 -> Fault Injection Lidar1/7
  Fault Injection Lidar1/3 -> Lidar Adapter1/4
  Fault Injection Lidar2/2 -> Lidar Adapter2/3
  Demux2/4 -> Fault Injection Listener Camera 2/5
  Fault Injection Lidar2/3 -> Lidar Adapter2/4
  MissionPlanning/1 -> ROS Send Simulink State/7
  Fault Injection Listener Lidar 3/1 -> Fault Injection Lidar2/5
  [gt_camera1_b] -> Fault Injection Camera1/3
  [gt_camera_tl_r] -> Fault Injection Camera2/1
  [lidar4_intensity] -> Fault Injection Lidar3/4
  [gt_camera1_g] -> Fault Injection Camera1/2
  Ssmp/1 -> ROS Send Simulink State/10
  FaultInjectionCamera2/1 -> Fault Injection Listener Camera 2/1
  Fault Injection Listener Lidar 1/5 -> Fault Injection Lidar/9
  Fault Injection Listener GNSS/2 -> Fault Injection GNSS/3
  Fault Injection Listener Lidar 2/2 -> Fault Injection Lidar1/6
  Demux/6 -> Fault Injection Listener Camera 1/7
  [fi_lidar_rain_a] -> Fault Injection Listener Lidar 1/5
  Fault Injection Listener Lidar 2/1 -> Fault Injection Lidar1/5
  Fault Injection Lidar/4 -> Lidar Adapter/5
  Fault Injection Listener Camera 1/1 -> Fault Injection Camera1/4
  Fault Injection Camera1/1 -> [camera1_r]
  [gt_camera2_b] -> Fault Injection Camera/3
  Fault Injection Camera/1 -> [camera2_r]
  [fi_lidar_rain_b] -> Fault Injection Listener Lidar 1/6
  [yaw_rate] -> ROS Send Velocity/2
  Demux2/6 -> Fault Injection Listener Camera 2/7
  FaultInjectionLidar3/1 -> Fault Injection Listener Lidar 3/1
  FaultInjectionCamera1/1 -> Fault Injection Listener Camera 1/1
  FaultInjectionLidar1/1 -> Fault Injection Listener Lidar 1/1
  Lidar Adapter3/1 -> [lidar4]
  [fi_lidar_range_variance] -> Fault Injection Listener Lidar 3/2
  Recording/1 -> ROS Send Simulink State/1
  MotionPlanning/1 -> ROS Send Simulink State/8
  FaultInjectionGNSS/1 -> Fault Injection Listener GNSS/1
  fi_lidar_rain_a/1 -> [fi_lidar_rain_a]
  fi_lidar_rain_reflectivity/1 -> [fi_lidar_rain_reflectivity]
  FakeLocalization/1 -> ROS Send Simulink State/5
  EnableSendVelocity/1 -> ROS Send Velocity/Enable
  FaultInjectionLidar4/1 -> Fault Injection Listener Lidar 4/1
  [lidar2] -> ROS Send Lidar/2
  [lidar4] -> ROS Send Lidar/4
  EnableSendCamera2/1 -> ROS Send Camera 2/Enable
  Fault Injection Listener TL Camera/5 -> Fault Injection Camera2/8
  [base_link_pose] -> Fault Injection GNSS/1
  EnableSendSwitch/1 -> ROS Send Switch Command/Enable
  EnableSendLidar/1 -> ROS Send Lidar/Enable
  Fault Injection Listener Camera 1/6 -> Fault Injection Camera1/9
  [lidar1] -> ROS Send Lidar/1
  [velocity] -> ROS Send Velocity/1
  Fault Injection Listener Lidar 4/5 -> Fault Injection Lidar3/9
  Initial checks/1 -> ROS send RCV states/1
  CoG offset z/1 -> Car_Pose1/9
  Switch/1 -> ROS Send Simulink State/9
  EnableSendGNSS/1 -> ROS Send GNSS/Enable
  Demux1/4 -> Fault Injection Listener TL Camera/5
  Fault Injection Lidar/2 -> Lidar Adapter/3
  OrientationLidar2/1 -> Lidar Adapter1/1
  Fault Injection Listener Lidar 2/5 -> Fault Injection Lidar1/9
  [radar_targetID] -> radarDetections/4
  [Roty] -> Car_Pose1/5
  [base_link_pose] -> ROS Send Odometry/1
  [yaw_rate] -> ROS Send Odometry/3
  Fault Injection Listener Lidar 4/6 -> Fault Injection Lidar3/10
  fi_lidar_rain_intensity/1 -> [fi_lidar_rain_intensity]
  Detection/1 -> ROS Send Simulink State/6
  [velocity] -> ROS Send Odometry/2
  EnableSendOdometry/1 -> ROS Send Odometry/Enable
  EnableSendCamera1/1 -> ROS Send Camera/Enable
  [gt_camera2_r] -> Fault Injection Camera/1
  Fault Injection Lidar/3 -> Lidar Adapter/4
  [Rotz] -> Car_Pose1/6
  fi_radar_theta_variance/1 -> [fi_radar_theta_variance]
  Car_Pose1/1 -> [base_link_pose]
  Fault Injection Listener Lidar 1/8 -> Fault Injection Lidar/12
  Bus Selector1/3 -> Fault Injection Radar/3  "<Phi[deg]>"
  [fi_lidar_rain_intensity] -> Fault Injection Listener Lidar 2/4
  Localization/1 -> ROS Send Simulink State/4
  [y] -> Car_Pose1/2
  [z] -> Car_Pose1/3
  Sensing/1 -> ROS Send Simulink State/3
  Fault Injection Listener Camera 2/4 -> Fault Injection Camera/7
  [x] -> Car_Pose1/1
  Bus Selector1/2 -> Fault Injection Radar/2  "<Theta[deg]>"
  Fault Injection Lidar2/1 -> Lidar Adapter2/2
  EnableSendRadar/1 -> radarDetections/Enable
  [fi_lidar_rain_a] -> Fault Injection Listener Lidar 3/5
  Bus Selector1/4 -> Fault Injection Radar/4  "<TargetTypeID[-]>"
  [lidar3_theta] -> Fault Injection Lidar2/2
  [fi_lidar_max_range] -> Fault Injection Listener Lidar 2/8
  Lidar Adapter/1 -> [lidar1]
  fi_lidar_rain_b/1 -> [fi_lidar_rain_b]
  [fi_lidar_rain_reflectivity] -> Fault Injection Listener Lidar 2/7
  FaultInjectionRadar/1 -> Fault Injection Listener Radar/1
  EnableSendClock/1 -> ROS Send Clock/Enable
  Fault Injection Listener Lidar 4/4 -> Fault Injection Lidar3/8
  Fault Injection Lidar3/4 -> Lidar Adapter3/5
  CoG offset x/1 -> Car_Pose1/7
  [lidar3] -> ROS Send Lidar/3
  Fault Injection Listener Lidar 2/6 -> Fault Injection Lidar1/10
  [fi_lidar_theta_variance] -> Fault Injection Listener Lidar 2/3
  [camera_tl_b] -> ROS Send Camera TL/3
  Bus Selector1/1 -> Fault Injection Radar/1  "<Range[m]>"
  [Roty] -> ROS Send IMU/2
  [lidar3_intensity] -> Fault Injection Lidar2/4
  Rviz/1 -> ROS Send Simulink State/11
  Fault Injection Listener GNSS/1 -> Fault Injection GNSS/2
  [camera1_g] -> ROS Send Camera/2
  Fault Injection Listener Lidar 1/7 -> Fault Injection Lidar/11
  Fault Injection Listener Camera 1/2 -> Fault Injection Camera1/5
  Lidar Adapter2/1 -> [lidar3]
  Fault/1 -> ROS send RCV states/3
  [fi_lidar_rain_reflectivity] -> Fault Injection Listener Lidar 3/7
  [Rotx] -> Car_Pose1/4
  fi_camera_patch_size_y/1 -> [fi_camera_patch_size_y]
  Fault Injection Lidar3/1 -> Lidar Adapter3/2
  SELF_Demux/4(rotx [deg]) -> [Rotx]
  SELF_Demux/6(rotz [deg]) -> [Rotz]
  SELF_Demux/3(z [m]) -> [z]
  SELF_Demux/12(yaw rate [deg/s]) -> [yaw_rate]
  SELF_Demux/10(velocity [m/s]) -> Dynamics_Empty/1(In1), [velocity]
  SELF_Demux/2(y [m]) -> [y]
  Radar_1_Demux/1(Radar Data) -> [gt_radar]
  SELF_Demux/5(roty [deg]) -> [Roty]
  SELF_Demux/1(x [m]) -> [x]
  PointCloudSensor_2_Angles_Demux/1(Theta) -> [lidar2_theta]
  PointCloudSensor_4_Angles_Demux/2(Phi) -> [lidar4_phi]
  PointCloudSensor_3_Angles_Demux/2(Phi) -> [lidar3_phi]
  PointCloudSensor_3_Intensity_Demux/1(Intensity) -> [lidar3_intensity]
  PointCloudSensor_3_Angles_Demux/1(Theta) -> [lidar3_theta]
  PointCloudSensor_3_Range_Demux/1(Range) -> [lidar3_range]
  PointCloudSensor_2_Range_Demux/1(Range) -> [lidar2_range]
  PointCloudSensor_4_Angles_Demux/1(Theta) -> [lidar4_theta]
  PointCloudSensor_2_Angles_Demux/2(Phi) -> [lidar2_phi]
  PointCloudSensor_1_Angles_Demux/1(Theta) -> [lidar1_theta]
  PointCloudSensor_1_Angles_Demux/2(Phi) -> [lidar1_phi]
  PointCloudSensor_1_Intensity_Demux/1(Intensity) -> [lidar1_intensity]
  PointCloudSensor_1_Range_Demux/1(Range) -> [lidar1_range]
  PointCloudSensor_2_Intensity_Demux/1(Intensity) -> [lidar2_intensity]
  PointCloudSensor_4_Range_Demux/1(Range) -> [lidar4_range]
  PointCloudSensor_4_Intensity_Demux/1(Intensity) -> [lidar4_intensity]
  Camera_2_CM_Demux/1(R) -> [gt_camera2_r], Camera_2_CM_Display/1
  Camera_2_CM_Demux/2(G) -> [gt_camera2_g], Camera_2_CM_Display/2
  Camera_tl_CM_Demux/3(B) -> [gt_camera_tl_b], Camera_tl_CM_Display/3
  Camera_1_CM_Demux/2(G) -> [gt_camera1_g], Camera_1_CM_Display/2
  Camera_tl_CM_Demux/2(G) -> [gt_camera_tl_g], Camera_tl_CM_Display/2
  Camera_2_CM_Demux/3(B) -> [gt_camera2_b], Camera_2_CM_Display/3
  Camera_1_CM_Demux/1(R) -> [gt_camera1_r], Camera_1_CM_Display/1
  Camera_tl_CM_Demux/1(R) -> [gt_camera_tl_r], Camera_tl_CM_Display/1
  Camera_1_CM_Demux/3(B) -> [gt_camera1_b], Camera_1_CM_Display/3
  STATE_BMW_X5_SUV_1_rc/1 -> STATE_BMW_X5_SUV_1_bus/1
  SELF_BMW_X5_SUV_1/1 -> SELF_Demux/1(SELF)
  Radar_1/1 -> Radar_1_Demux/1(Radar)
  PointCloudSensor_1/1 -> PointCloudSensor_1_Range_Demux/1(In1), PointCloudSensor_1_Angles_Demux/1(In2), PointCloudSensor_1_Intensity_Demux/1(In1)
  PointCloudSensor_2/1 -> PointCloudSensor_2_Range_Demux/1(In1), PointCloudSensor_2_Angles_Demux/1(In2), PointCloudSensor_2_Intensity_Demux/1(In1)
  PointCloudSensor_3/1 -> PointCloudSensor_3_Range_Demux/1(In1), PointCloudSensor_3_Angles_Demux/1(In2), PointCloudSensor_3_Intensity_Demux/1(In1)
  PointCloudSensor_4/1 -> PointCloudSensor_4_Range_Demux/1(In1), PointCloudSensor_4_Angles_Demux/1(In2), PointCloudSensor_4_Intensity_Demux/1(In1)
  Camera_1/1 -> Camera_1_CM_Demux/1(In1)
  Camera_tl/1 -> Camera_tl_CM_Demux/1(In1)
  Camera_2/1 -> Camera_2_CM_Demux/1(In1)
  Dynamics_Empty/1(State) -> STATE_BMW_X5_SUV_1_rc/1
  SELF_Demux/7(GPS lat [deg]) -> Terminator_1/1
  SELF_Demux/8(GPS long [deg]) -> Terminator_2/1
  SELF_Demux/9(GPS alt [m]) -> Terminator_3/1
  SELF_Demux/11(heading [deg]) -> Terminator_4/1

== system W06_Tiny_Town_cs/Camera_1 ==
  Sensor : S-Function  FunctionName=sfun_Camera  Parameters=sensorID, dataWidth, dataHeight, channelsPerImage, numberOfImages, timestep  SFunctionDeploymentMode=off  EnableBusSupport=off  mask(PreScan Source Block: Camera Sensor){sensorID=27933, dataWidth=720, dataHeight=2880, channelsPerImage=3, numberOfImages=1, timestep=1/20}
      mask prompts: sensorID "Sensor ID"; dataWidth "Data width"; dataHeight "Data Height"; channelsPerImage "Channels per image"; numberOfImages "Number of images"; timestep "MATLAB timestep:"
      mask help: The Camera Sensor provides a color or monochrome image.
      mask Help: eval('openHelp(457)')
      mask Display: image(imread('CameraSensor.png'))
  Camera_1 : Outport  Tag=outport/Camera/CameraSensor  OutDataTypeStr=uint8  SampleTime=1/20
  wires:
  Sensor/1 -> Camera_1/1

== system W06_Tiny_Town_cs/Camera_2 ==
  Sensor : S-Function  FunctionName=sfun_Camera  Parameters=sensorID, dataWidth, dataHeight, channelsPerImage, numberOfImages, timestep  SFunctionDeploymentMode=off  EnableBusSupport=off  mask(PreScan Source Block: Camera Sensor){sensorID=27937, dataWidth=720, dataHeight=2880, channelsPerImage=3, numberOfImages=1, timestep=1/20}
      mask prompts: sensorID "Sensor ID"; dataWidth "Data width"; dataHeight "Data Height"; channelsPerImage "Channels per image"; numberOfImages "Number of images"; timestep "MATLAB timestep:"
      mask help: The Camera Sensor provides a color or monochrome image.
      mask Help: eval('openHelp(457)')
      mask Display: image(imread('CameraSensor.png'))
  Camera_2 : Outport  Tag=outport/Camera/CameraSensor  OutDataTypeStr=uint8  SampleTime=1/20
  wires:
  Sensor/1 -> Camera_2/1

== system W06_Tiny_Town_cs/Camera_tl ==
  Sensor : S-Function  FunctionName=sfun_Camera  Parameters=sensorID, dataWidth, dataHeight, channelsPerImage, numberOfImages, timestep  SFunctionDeploymentMode=off  EnableBusSupport=off  mask(PreScan Source Block: Camera Sensor){sensorID=27934, dataWidth=720, dataHeight=2880, channelsPerImage=3, numberOfImages=1, timestep=1/20}
      mask prompts: sensorID "Sensor ID"; dataWidth "Data width"; dataHeight "Data Height"; channelsPerImage "Channels per image"; numberOfImages "Number of images"; timestep "MATLAB timestep:"
      mask help: The Camera Sensor provides a color or monochrome image.
      mask Help: eval('openHelp(457)')
      mask Display: image(imread('CameraSensor.png'))
  Camera_tl : Outport  Tag=outport/Camera/CameraSensor  OutDataTypeStr=uint8  SampleTime=1/20
  wires:
  Sensor/1 -> Camera_tl/1
